simulink model "PID_VELOCIDAD_MOTORDC_ANTI_WINDUP"  (R2023a)
settings: Solver=ode1  StartTime=0.0  StopTime=inf  FixedStep=0.01  RelTol=1e-3
libraries: arduinolib x3, arduinosensorlib x1, simulink x1
settings Model: ExtModeTrigDuration=2  Creator=Mario  LastModifiedBy=Mario
settings OptimizationCC: EnhancedBackFolding=on  PassReuseOutputArgsAs=Individual arguments  ZeroExternalMemoryAtStartup=off  ZeroInternalMemoryAtStartup=off  MaxStackSize=64  OptimizeBlockOrder=speed  DifferentSizesBufferReuse=on  OptimizationCustomize=off  EfficientTunableParamExpr=on
settings DebuggingCC: ParameterTunabilityLossMsg=error
settings HardwareCC: ProdBitPerPointer=32  ProdBitPerSizeT=32  ProdBitPerPtrDiffT=32  ProdLargestAtomicInteger=Long  ProdLargestAtomicFloat=Double  ProdWordSize=32  ProdHWDeviceType=ARM Compatible->ARM Cortex  UseEmbeddedCoderFeatures=off
settings SFSimCC: MATLABDynamicMemAlloc=off
settings RTWCC: Description=Embedded Coder  SystemTargetFile=ert.tlc  HardwareBoard=Arduino Due  TemplateMakefile=ert_default_tmf  Toolchain=Arduino ARM  BuildConfiguration=Faster Runs
settings CodeAppCC: ForceParamTrailComments=on  IgnoreCustomStorageClasses=off  OperatorAnnotations=on  SimulinkDataObjDesc=on  SFDataObjDesc=on  InsertBlockDesc=on
settings ERTTargetCC: SupportContinuousTime=on  SupportNonInlinedSFcns=on  SupportVariableSizeSignals=on  ExtModeTransport=3  ExtModeStaticAlloc=on  ExtModeAutomaticAllocSize=off  ExtModeStaticAllocSize=24576  ExtModeMexFile=ext_xcp  ExtModeIntrfLevel=Level2 - Open

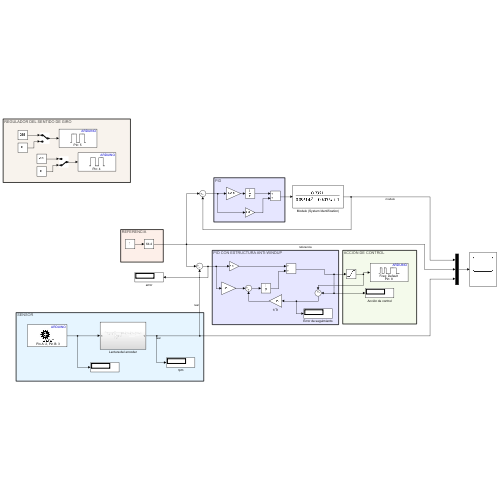
[thumbnail: Simulink's stored preview of the top-level diagram]
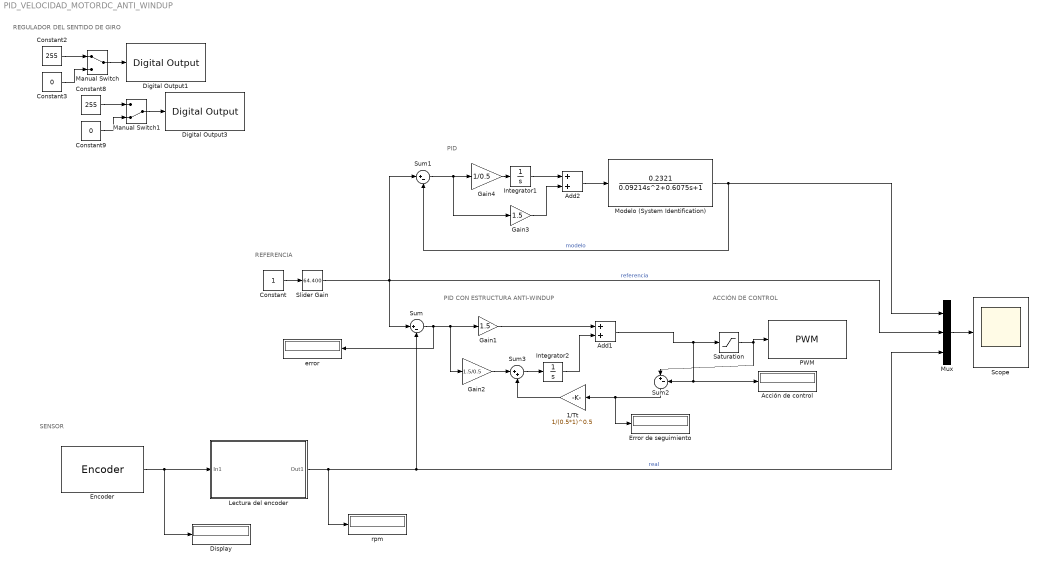
== system PID_VELOCIDAD_MOTORDC_ANTI_WINDUP ==
  note: SENSOR
  note: REFERENCIA
  note: ACCIÓN DE CONTROL
  note: REGULADOR DEL SENTIDO DE GIRO
  note: PID
  note: PID CON ESTRUCTURA ANTI-WINDUP
  1/Tt : Gain  Gain=1/(0.5*1)^0.5
  Acción de control : Display
  Add1 : Sum
  Add2 : Sum
  Constant : Constant
  Constant2 : Constant  Value=255
  Constant3 : Constant  Value=0
  Constant8 : Constant  Value=255
  Constant9 : Constant  Value=0
  Digital Output1 : arduinolib/Digital Output  pinNumber=5  Direction=output  blockPlatform=arduino
  Digital Output3 : arduinolib/Digital Output  pinNumber=4  Direction=output  blockPlatform=arduino
  Display : Display
  Encoder : arduinosensorlib/Encoder  InputA=2  InputB=3  Mode=No reset  SampleTime=-1
  Error de seguimiento : Display
  Gain1 : Gain  Gain=1.5
  Gain2 : Gain  Gain=1.5/0.5
  Gain3 : Gain  Gain=1.5
  Gain4 : Gain  Gain=1/0.5
  Integrator1 : Integrator
  Integrator2 : Integrator
  Lectura del encoder : Subsystem
  Manual Switch : ManualSwitch
  Manual Switch1 : ManualSwitch  CurrentSetting=0
  Modelo (System Identification) : TransferFcn  Numerator=[0.2321]  Denominator=[0.09214 0.6075 1]
  Mux : Mux  Inputs=3
  PWM : arduinolib/PWM  pinNumber=8  frequencyType=Default  desiredFrequency=490.2  achievableFrequency=490.2
  Saturation : Saturate  UpperLimit=255  LowerLimit=0
  Scope : Scope
  Slider Gain : simulink/Math Operations/Slider Gain  gain=64.400  low=0  high=70
  Sum : Sum  Inputs=|+-
  Sum1 : Sum  Inputs=|+-
  Sum2 : Sum  Inputs=|+-
  Sum3 : Sum  Inputs=|++
  error : Display
  rpm : Display
  wires:
  Constant3/1 -> Manual Switch/2
  Constant8/1 -> Manual Switch1/1
  Constant9/1 -> Manual Switch1/2
  Constant2/1 -> Manual Switch/1
  Manual Switch/1 -> Digital Output1/1
  Manual Switch1/1 -> Digital Output3/1
  Lectura del encoder/1(Out1) -> Sum/2, Mux/3, rpm/1  "real"
  Encoder/1 -> Display/1, Lectura del encoder/1(In1)
  Add1/1 -> Saturation/1, Acción de control/1, Sum2/2
  Saturation/1 -> PWM/1, Sum2/1
  Slider Gain/1 -> Mux/2, Sum/1, Sum1/1  "referencia"
  Mux/1 -> Scope/1
  Sum1/1 -> Gain3/1, Gain4/1
  Gain4/1 -> Integrator1/1
  Gain3/1 -> Add2/2
  Integrator1/1 -> Add2/1
  Add2/1 -> Modelo (System Identification)/1
  Modelo (System Identification)/1 -> Mux/1, Sum1/2  "modelo"
  Gain1/1 -> Add1/1
  Gain2/1 -> Sum3/1
  Sum/1 -> error/1, Gain2/1, Gain1/1
  Sum2/1 -> Error de seguimiento/1, 1/Tt/1
  Sum3/1 -> Integrator2/1
  Integrator2/1 -> Add1/2
  1/Tt/1 -> Sum3/2
  Constant/1 -> Slider Gain/1

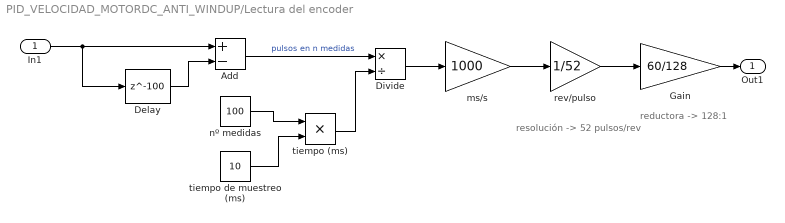
== system PID_VELOCIDAD_MOTORDC_ANTI_WINDUP/Lectura del encoder ==
  note: reductora -> 128:1
  note: resolución -> 52 pulsos/rev
  In1 : Inport
  Add : Sum  Inputs=+-
  Delay : Delay  DelayLength=100
  Divide : Product  Inputs=*/
  Gain : Gain  Gain=60/128
  ms/s : Gain  Gain=1000
  nº medidas : Constant  Value=100
  rev/pulso : Gain  Gain=1/52
  tiempo (ms) : Product  Inputs=**
  tiempo de muestreo (ms) : Constant  Value=10
  Out1 : Outport
  wires:
  Delay/1 -> Add/2
  Divide/1 -> ms/s/1
  In1/1 -> Delay/1, Add/1
  nº medidas/1 -> tiempo (ms)/1
  Add/1 -> Divide/1  "pulsos en n medidas"
  rev/pulso/1 -> Gain/1
  Gain/1 -> Out1/1
  ms/s/1 -> rev/pulso/1
  tiempo de muestreo (ms)/1 -> tiempo (ms)/2
  tiempo (ms)/1 -> Divide/2
